simulink model "pendulum_control"  (R2018b)
settings: Solver=VariableStepAuto  StartTime=0.0  StopTime=10.0  RelTol=1e-3
values from neighbouring files (symbols this model uses):
  alpha = 0.9    [inverted_pendulum_final.m]
undefined symbols (not defined in the file or in its folder): K, Ki
settings Model: Creator=ipebo  LastModifiedBy=ipebo

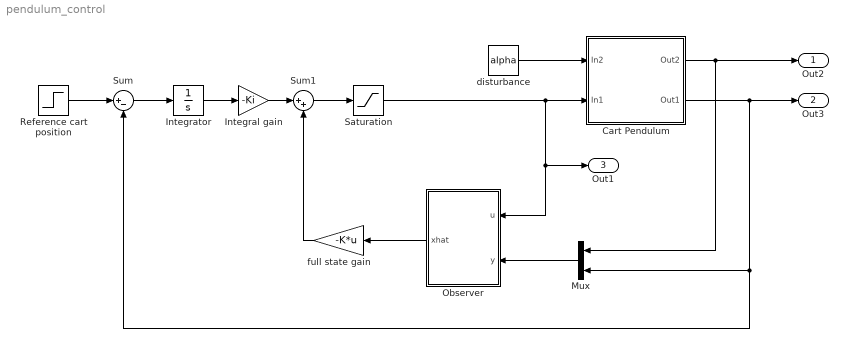
== system pendulum_control ==
  Cart Pendulum : Subsystem
  Integral gain : Gain  Gain=-Ki
  Integrator : Integrator
  Mux : Mux  Inputs=2
  Observer : Subsystem
  Reference cart position : Step  SampleTime=0
  Saturation : Saturate
  Sum : Sum  Inputs=|+-
  Sum1 : Sum  Inputs=|++
  disturbance : Constant  Value=alpha
  full state gain : Gain  Gain=-K*u
  Out2 : Outport  SignalName=theta(t)
  Out3 : Outport  Port=2  SignalName=s(t)
  Out1 : Outport  Port=3  SignalName=a(t)
  wires:
  Reference cart position/1 -> Sum/1
  Sum/1 -> Integrator/1
  Integrator/1 -> Integral gain/1
  Integral gain/1 -> Sum1/1
  Sum1/1 -> Saturation/1
  full state gain/1 -> Sum1/2
  Saturation/1 -> Out1/1, Observer/1(u), Cart Pendulum/2(In1)
  Observer/1(xhat) -> full state gain/1
  disturbance/1 -> Cart Pendulum/1(In2)
  Cart Pendulum/1(Out2) -> Out2/1, Mux/1
  Mux/1 -> Observer/2(y)
  Cart Pendulum/2(Out1) -> Out3/1, Sum/2, Mux/2

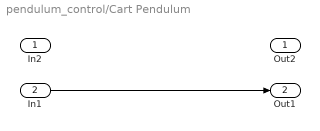
== system pendulum_control/Cart Pendulum ==
  In2 : Inport
  In1 : Inport  Port=2
  Out2 : Outport
  Out1 : Outport  Port=2
  wires:
  In1/1 -> Out1/1

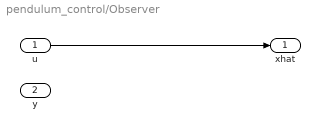
== system pendulum_control/Observer ==
  u : Inport
  y : Inport  Port=2
  xhat : Outport
  wires:
  u/1 -> xhat/1
